simulink model "Reciever"  (R2023b)
settings: Solver=FixedStepAuto  StartTime=0.0  StopTime=10.0  RelTol=1e-3
undefined symbols (not defined in the file): Data_Display, Data_Input, reciever0x5B10x5D
libraries: androiduilib x2, androidaudiovideolib x1, androidcommunicationlib x1
settings Model: Creator=Parth Dembla  LastModifiedBy=Swayam
settings OptimizationCC: EnhancedBackFolding=on  PassReuseOutputArgsAs=Individual arguments  ZeroExternalMemoryAtStartup=off  ZeroInternalMemoryAtStartup=off  MaxStackSize=64  OptimizeBlockOrder=speed  DifferentSizesBufferReuse=on  OptimizationCustomize=off  EfficientTunableParamExpr=on
settings DebuggingCC: ParameterTunabilityLossMsg=error  IntegerSaturationMsg=none
settings HardwareCC: ProdBitPerLong=64  ProdLargestAtomicInteger=LongLong  ProdLargestAtomicFloat=Double  ProdLongLongMode=on  ProdHWDeviceType=ARM Compatible->ARM 64-bit (LP64)
settings SFSimCC: MATLABDynamicMemAlloc=off
settings RTWCC: Description=Embedded Coder  SystemTargetFile=ert.tlc  HardwareBoard=Android Device (64bit)  TLCOptions="-aInlineSetEventsForThisBaseRateFcn=TLC_FALSE -aSuppressMultiTaskScheduler=TLC_FALSE  -aRateBasedStepFcn=0"  TemplateMakefile=ert_default_tmf  RTWVerbose=off  Toolchain=Android SDK/NDK Tools
settings CodeAppCC: ForceParamTrailComments=on  IgnoreCustomStorageClasses=off  OperatorAnnotations=on  SimulinkDataObjDesc=on  SFDataObjDesc=on  InsertBlockDesc=on

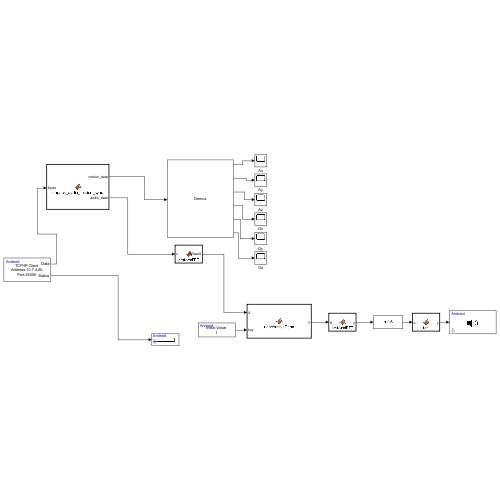
[thumbnail: Simulink's stored preview of the top-level diagram]
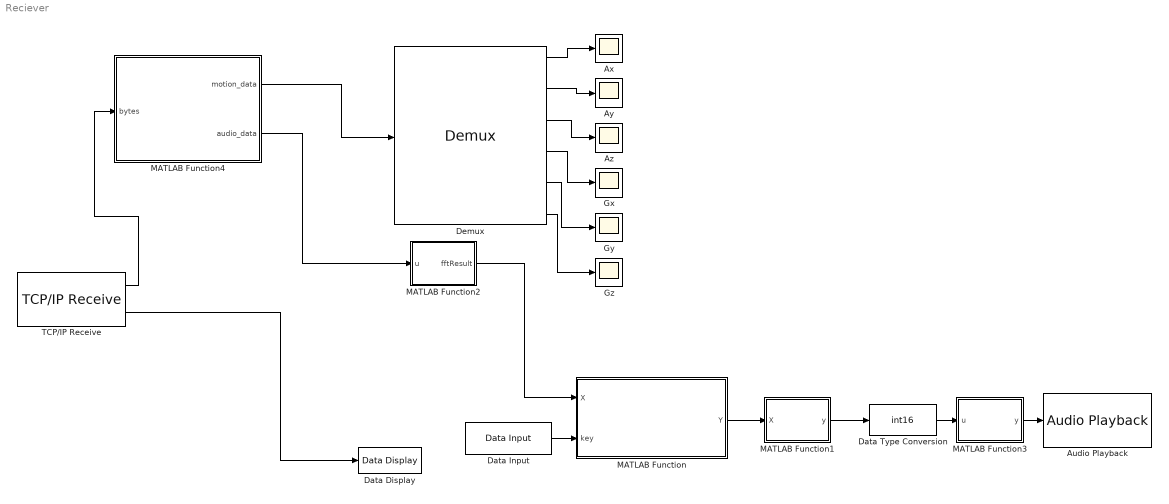
== system Reciever ==
  Audio Playback : androidaudiovideolib/Audio Playback  SampleFreq=44100  AudioSamplingFreq=44100  SampleTime=0.1  DeviceStr=0  QueueDuration=0  BlockPlatform=Android
  Ax : Scope
  Ay : Scope
  Az : Scope
  Data Display : androiduilib/Data Display  DataDisplayId=reciever0x5B10x5D/Data_Display  Format=Float  Precision=6  SimulateUsing=Code generation  blockPlatform=Android
  Data Input : androiduilib/Data Input  isCharVector=off  Value=1.0  CharVector=Hello World  OutputDataType=int16  maxCharVectorSize=100  DataInputId=reciever0x5B10x5D/Data_Input  SampleTime=0.1
  Data Type Conversion : DataTypeConversion  OutDataTypeStr=int16  SaturateOnIntegerOverflow=off  RndMeth=Floor
  Demux : Demux  Outputs=6
      settings: DisplayOption=none
  Gx : Scope
  Gy : Scope
  Gz : Scope
  MATLAB Function : MATLAB Function  TreatAsAtomicUnit=on
  MATLAB Function1 : MATLAB Function  TreatAsAtomicUnit=on
  MATLAB Function2 : MATLAB Function  TreatAsAtomicUnit=on
  MATLAB Function3 : MATLAB Function  TreatAsAtomicUnit=on
  MATLAB Function4 : MATLAB Function  TreatAsAtomicUnit=on
  TCP/IP Receive : androidcommunicationlib/TCP//IP Receive  TCPReceiveId=reciever0x5B10x5D/TCP//IP_Receive  Mode_=Client  LocalServerPort_=25000  RemoteAddr_=10.7.4.60  RemoteServerPort_=25000  DataType_=uint8  DataSize_=8848  SampleTime_=0.1  ClientPortBindingSelection_=off  ClientPortToBind_=35000  BlockingMode_=on  BlockTimeout_=0.1
  wires:
  MATLAB Function/1(Y) -> MATLAB Function1/1(X)
  MATLAB Function2/1(fftResult) -> MATLAB Function/1(X)
  TCP/IP Receive/2 -> Data Display/1
  MATLAB Function3/1(y) -> Audio Playback/1
  MATLAB Function1/1(y) -> Data Type Conversion/1
  Data Type Conversion/1 -> MATLAB Function3/1(u)
  Data Input/1 -> MATLAB Function/2(key)
  TCP/IP Receive/1 -> MATLAB Function4/1(bytes)
  MATLAB Function4/2(audio_data) -> MATLAB Function2/1(u)
  MATLAB Function4/1(motion_data) -> Demux/1
  Demux/1 -> Ax/1
  Demux/2 -> Ay/1
  Demux/3 -> Az/1
  Demux/4 -> Gx/1
  Demux/5 -> Gy/1
  Demux/6 -> Gz/1

== matlab function Reciever/MATLAB Function ==
  data: X input; Y output; key input
function Y = unscramblePerm(X, key)

[N,C] = size(X);
Y = complex(zeros(N,C,'like',X));



posIdx = 2:N/2;
negIdx = N - posIdx + 2;
K = numel(posIdx);  if K==0, Y = X; return; end


state = hash_fxn(uint8(key));
state = bitxor(state, uint32(N));
if state==0, state = uint32(1); end
perm = scrambling(state, K);


invp = zeros(1,K,'uint32');
for i = 1:K
    invp(perm(i)) = uint32(i);
end

Y(posIdx,:)      = X(posIdx(invp),:);
Y(negIdx,:)      = conj(Y(posIdx,:));
Y([1, N/2+1], :) = X([1, N/2+1], :);
end

function seed = hash_fxn(keyBytes)
b0=uint32(0); b1=uint32(0); b2=uint32(0); b3=uint32(0);
if numel(keyBytes)>=1, b0 = uint32(keyBytes(1)); end
if numel(keyBytes)>=2, b1 = bitshift(uint32(keyBytes(2)),  8); end
if numel(keyBytes)>=3, b2 = bitshift(uint32(keyBytes(3)), 16); end
if numel(keyBytes)>=4, b3 = bitshift(uint32(keyBytes(4)), 24); end
seed = bitor(bitor(b0,b1), bitor(b2,b3));
if seed==0, seed = uint32(1); end
end

function perm = scrambling(state, K)
perm = 1:K;
for i = K:-1:2
    [state, r] = xorshift32(state);
    j = double(bitshift(uint64(r)*uint64(i), -32)) + 1;  % 1..i
    t = perm(i); perm(i) = perm(j); perm(j) = t;
end



function [state, r] = xorshift32(state)

state = bitxor(state, bitshift(state, 13));
state = bitxor(state, bitshift(state, -17));
state = bitxor(state, bitshift(state, 5));
r = state;  % uint32
end
end

== matlab function Reciever/MATLAB Function2 ==
  data: u input; fftResult output
function fftResult = performFFT(u)
    fftResult=fft(u);
end

== matlab function Reciever/MATLAB Function3 ==
  data: u input; y output
function y = fcn(u)

y = [u,u];

== matlab function Reciever/MATLAB Function4 ==
  data: bytes input; motion_data output; audio_data output
function [motion_data, audio_data] = unpack_audio_motion_sync(bytes)
                 
motion_data   = zeros(1,6,'single');         % 1x6
audio_data = zeros(4410,1,'int16');       % 4410x1





motion_data(1,1:6)  = typecast(bytes(5:28), 'single').';   % 6 singles
audio_data(:,1)  = typecast(bytes(29:8848), 'int16');   % 4410 samples
end

== matlab function Reciever/MATLAB Function1 ==
  data: X input; y output
function y = performIFFT(X)
% X: N×C complex two-sided spectrum (N even, DC at 1, Nyquist at N/2+1)
% y: N×C real double time-domain frame
%#codegen
Xc = complex(double(X));
N  = size(Xc,1);
y  = real(ifft(Xc,N,1));
end
